simulink model "FAULT_MANAGEMENT"  (R2024b)
settings: configuration reference "MODEL_CONFIG_CHILD" (kept outside this file)
undefined symbols (not defined in the file): BATTERY_UV_LIM_U16, BATTERY_UV_RST_LIM_U16, BOOLEAN_ONE, CURR_CUTOFF_CTR_U16, CURRENTCUTOFF_LIM_mA_i32, DEFAULT_SPD_LIM_U16, MILLI_SEC_COUNTS_3000_U16, MILLI_SEC_COUNTS_5000_U16, MOTOR_BLOCK_CTR_U16, SAMPLE_TIME_1MS, THROTT_ERR_LWRTHSD_U16, THROTT_ERR_UPRTHSD_U16, THROTTLE_INITIATION_VALUE_U16, ZERO_i32, ZERO_U16
libraries: simulink x11
settings Model: DataDictionary=MCU_FOC_MAIN_DD.sldd  EnableAccessToBaseWorkspace=off  Creator=415  LastModifiedBy=415
settings ConfigSetRef: SourceName=MODEL_CONFIG_CHILD

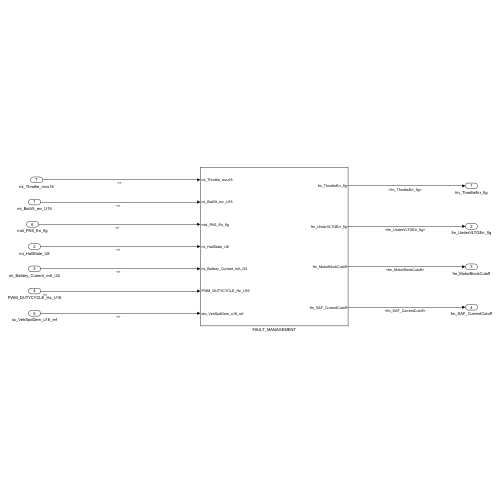
[thumbnail: Simulink's stored preview of the top-level diagram]
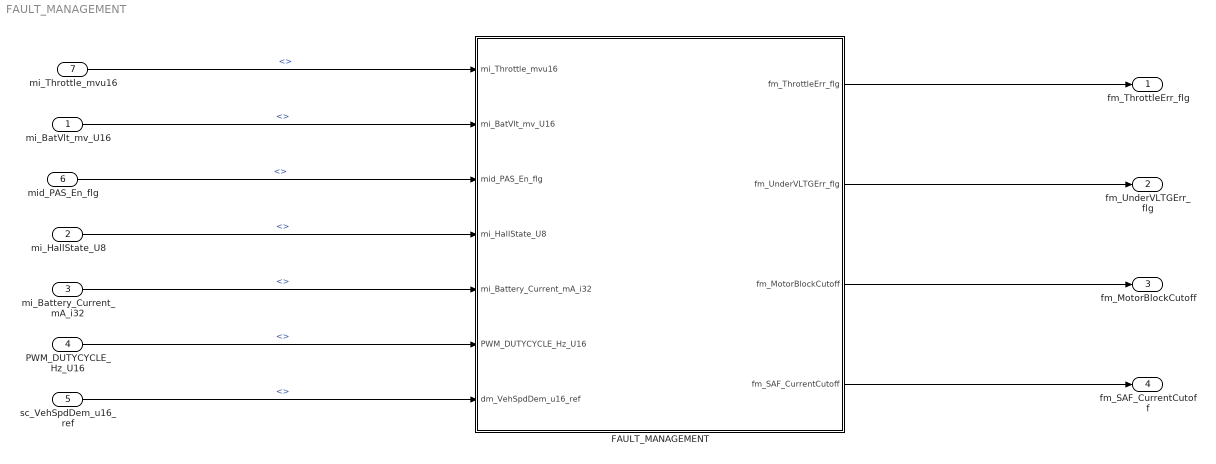
== system FAULT_MANAGEMENT ==
  mi_BatVlt_mv_U16 : Inport
  mi_HallState_U8 : Inport  Port=2
  mi_Battery_Current_mA_i32 : Inport  Port=3
  PWM_DUTYCYCLE_Hz_U16 : Inport  Port=4
  sc_VehSpdDem_u16_ref : Inport  Port=5
  mid_PAS_En_flg : Inport  Port=6
  mi_Throttle_mvu16 : Inport  Port=7
  FAULT_MANAGEMENT : Subsystem
  fm_ThrottleErr_flg : Outport
  fm_UnderVLTGErr_flg : Outport  Port=2
  fm_MotorBlockCutoff : Outport  Port=3
  fm_SAF_CurrentCutoff : Outport  Port=4
  wires:
  mi_Throttle_mvu16/1 -> FAULT_MANAGEMENT/1(mi_Throttle_mvu16)  "<>"
  sc_VehSpdDem_u16_ref/1 -> FAULT_MANAGEMENT/7(dm_VehSpdDem_u16_ref)  "<>"
  mi_BatVlt_mv_U16/1 -> FAULT_MANAGEMENT/2(mi_BatVlt_mv_U16)  "<>"
  FAULT_MANAGEMENT/1(fm_ThrottleErr_flg) -> fm_ThrottleErr_flg/1
  FAULT_MANAGEMENT/4(fm_SAF_CurrentCutoff) -> fm_SAF_CurrentCutoff/1
  mid_PAS_En_flg/1 -> FAULT_MANAGEMENT/3(mid_PAS_En_flg)  "<>"
  FAULT_MANAGEMENT/2(fm_UnderVLTGErr_flg) -> fm_UnderVLTGErr_flg/1
  FAULT_MANAGEMENT/3(fm_MotorBlockCutoff) -> fm_MotorBlockCutoff/1
  mi_Battery_Current_mA_i32/1 -> FAULT_MANAGEMENT/5(mi_Battery_Current_mA_i32)  "<>"
  PWM_DUTYCYCLE_Hz_U16/1 -> FAULT_MANAGEMENT/6(PWM_DUTYCYCLE_Hz_U16)  "<>"
  mi_HallState_U8/1 -> FAULT_MANAGEMENT/4(mi_HallState_U8)  "<>"

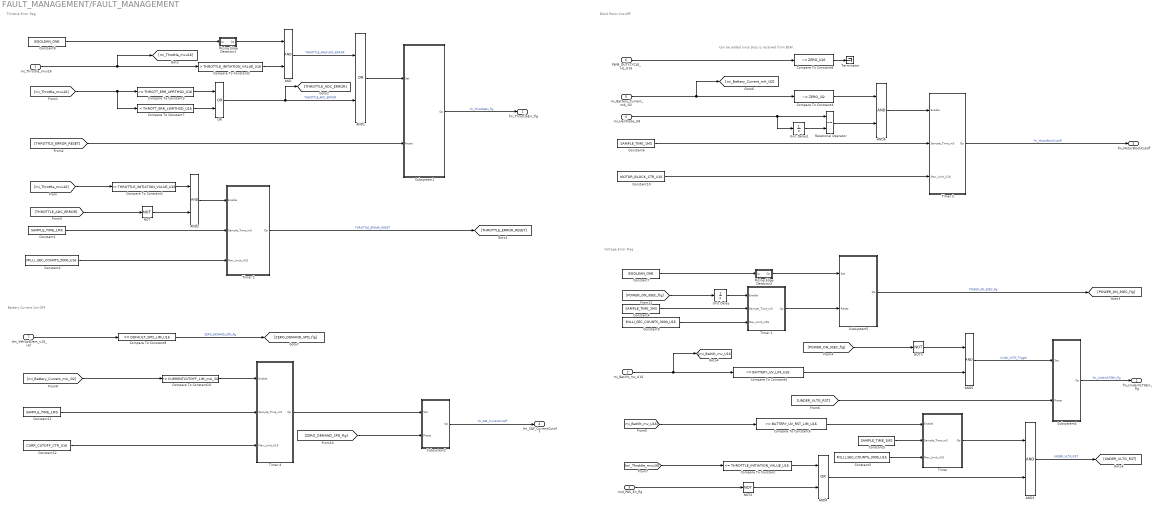
== system FAULT_MANAGEMENT/FAULT_MANAGEMENT ==
  note: Battery Current Cut-OFF
  note: Can be added once Duty is received from BSW.
  note: Block Rotor Cut-OFF
  note: Voltage Error Flag
  note: Throttle Error flag
  mi_Throttle_mvu16 : Inport
  mi_BatVlt_mv_U16 : Inport  Port=2
  mid_PAS_En_flg : Inport  Port=3
  mi_HallState_U8 : Inport  Port=4
  mi_Battery_Current_mA_i32 : Inport  Port=5
  PWM_DUTYCYCLE_Hz_U16 : Inport  Port=6
  dm_VehSpdDem_u16_ref : Inport  Port=7
  AND{,2..3,5..6} (5 alike) : Logic  AllPortsSameDT=off  OutDataTypeStr=boolean
  AND1 : Logic  Operator=OR  AllPortsSameDT=off  OutDataTypeStr=boolean
  AND4 : Logic  Operator=OR  AllPortsSameDT=off  OutDataTypeStr=boolean
  Compare To Constant : simulink/Logic and Bit Operations/Compare To Constant  relop=<=  const=THROTTLE_INITIATION_VALUE_U16  OutDataTypeStr=boolean
  Compare To Constant1 : simulink/Logic and Bit Operations/Compare To Constant  relop=<=  const=THROTTLE_INITIATION_VALUE_U16  OutDataTypeStr=boolean
  Compare To Constant10 : simulink/Logic and Bit Operations/Compare To Constant  relop=>=  const=CURRENTCUTOFF_LIM_mA_i32  OutDataTypeStr=boolean
  Compare To Constant2 : simulink/Logic and Bit Operations/Compare To Constant  relop=>  const=THROTTLE_INITIATION_VALUE_U16  OutDataTypeStr=boolean
  Compare To Constant3 : simulink/Logic and Bit Operations/Compare To Constant  relop=>=  const=THROTT_ERR_UPRTHSD_U16  OutDataTypeStr=boolean
  Compare To Constant4 : simulink/Logic and Bit Operations/Compare To Constant  relop=~=  const=ZERO_i32  OutDataTypeStr=boolean
  Compare To Constant5 : simulink/Logic and Bit Operations/Compare To Constant  relop=<=  const=BATTERY_UV_LIM_U16  OutDataTypeStr=boolean
  Compare To Constant6 : simulink/Logic and Bit Operations/Compare To Constant  relop=>=  const=BATTERY_UV_RST_LIM_U16  OutDataTypeStr=boolean
  Compare To Constant7 : simulink/Logic and Bit Operations/Compare To Constant  relop=<  const=THROTT_ERR_LWRTHSD_U16  OutDataTypeStr=boolean
  Compare To Constant8 : simulink/Logic and Bit Operations/Compare To Constant  relop=~=  const=ZERO_U16  OutDataTypeStr=boolean
  Compare To Constant9 : simulink/Logic and Bit Operations/Compare To Constant  relop===  const=DEFAULT_SPD_LIM_U16  OutDataTypeStr=boolean
  Constant{1,4..6,11} (5 alike) : Constant  Value=SAMPLE_TIME_1MS
  Constant10 : Constant  Value=MOTOR_BLOCK_CTR_U16
  Constant12 : Constant  Value=CURR_CUTOFF_CTR_U16
  Constant2 : Constant  Value=MILLI_SEC_COUNTS_5000_U16
  Constant3 : Constant  Value=MILLI_SEC_COUNTS_3000_U16
  Constant7 : Constant  Value=BOOLEAN_ONE
  Constant8 : Constant  Value=BOOLEAN_ONE
  Constant9 : Constant  Value=MILLI_SEC_COUNTS_3000_U16
  NOT : Logic  Operator=NOT  IconShape=distinctive  AllPortsSameDT=off  OutDataTypeStr=boolean
  NOT2 : Logic  Operator=NOT  IconShape=distinctive  AllPortsSameDT=off  OutDataTypeStr=boolean
  NOT3 : Logic  Operator=NOT  IconShape=distinctive  AllPortsSameDT=off  OutDataTypeStr=boolean
  OR : Logic  Operator=OR  AllPortsSameDT=off  OutDataTypeStr=boolean
  Relational Operator : RelationalOperator  Operator===  OutDataTypeStr=boolean  RndMeth=Simplest  InputSameDT=off
  Rising Edge Detector1 : Subsystem
  Rising Edge Detector2 : Subsystem
  Subsystem1 : Subsystem
  Subsystem2 : Subsystem
  Subsystem4 : Subsystem
  Subsystem5 : Subsystem
  Terminator : Terminator
  "Timer " : Subsystem
  Timer 1 : Subsystem
  Timer 2 : Subsystem
  Timer 3 : Subsystem
  Timer 4 : Subsystem
  Unit Delay : UnitDelay  SampleTime=-1  HasFrameUpgradeWarning=on
  Unit Delay1 : UnitDelay  SampleTime=-1  HasFrameUpgradeWarning=on
  fm_ThrottleErr_flg : Outport
  fm_UnderVLTGErr_flg : Outport  Port=2
  fm_MotorBlockCutoff : Outport  Port=3  OutputWhenDisabled=reset  InitialOutput=0
  fm_SAF_CurrentCutoff : Outport  Port=4  OutputWhenDisabled=reset  InitialOutput=0
  wires:
  Constant8/1 -> Rising Edge Detector1/1(Ip)
  mi_Throttle_mvu16/1 -> Compare To Constant2/1, [mi_Throttle_mvu16]
  Compare To Constant2/1 -> AND/2
  Rising Edge Detector1/1(Op) -> AND/1
  AND/1 -> AND1/1  "THROTTLE_MALFUNC_ERROR"
  Timer 2/1(Op) -> [THROTTLE_ERROR_RESET]  "THROTTLE_ERROR_RESET"
  Constant1/1 -> Timer 2/2(Sample_Time_mS)
  Compare To Constant1/1 -> AND2/1
  [mi_Throttle_mvu16] -> Compare To Constant1/1
  Constant2/1 -> Timer 2/3(Max_Limit_U16)
  Subsystem1/1(Op) -> fm_ThrottleErr_flg/1  "fm_ThrottleErr_flg"
  Compare To Constant7/1 -> OR/2
  Compare To Constant3/1 -> OR/1
  [THROTTLE_ERROR_RESET] -> Subsystem1/2(Reset)
  AND1/1 -> Subsystem1/1(Set)
  [mi_Throttle_mvu16] -> Compare To Constant3/1, Compare To Constant7/1
  OR/1 -> [THROTTLE_ADC_ERROR], AND1/2  "THROTTLE_ADC_ERROR"
  [THROTTLE_ADC_ERROR] -> NOT/1
  NOT/1 -> AND2/2
  AND2/1 -> Timer 2/1(Enable)
  Unit Delay/1 -> Timer 1/1(Enable)
  NOT3/1 -> AND5/1
  NOT2/1 -> AND4/2
  Subsystem5/1(Op) -> [POWER_ON_3SEC_flg]  "POWER_ON_3SEC_flg"
  Subsystem4/1(Op) -> fm_UnderVLTGErr_flg/1  "fm_UnderVLTGErr_flg"
  Compare To Constant5/1 -> AND5/2
  mid_PAS_En_flg/1 -> NOT2/1
  [mi_Throttle_mvu16] -> Compare To Constant/1
  Constant9/1 -> Timer 1/3(Max_Limit_U16)
  Constant4/1 -> Timer 1/2(Sample_Time_mS)
  Constant5/1 -> "Timer "/2(Sample_Time_mS)
  Rising Edge Detector2/1(Op) -> Subsystem5/1(Set)
  Compare To Constant6/1 -> "Timer "/1(Enable)
  Compare To Constant/1 -> AND4/1
  [POWER_ON_3SEC_flg] -> Unit Delay/1
  Constant7/1 -> Rising Edge Detector2/1(Ip)
  AND5/1 -> Subsystem4/1(Set)  "Under_VLTG_Trigger"
  mi_BatVlt_mv_U16/1 -> [mi_BatVlt_mv_U16], Compare To Constant5/1
  "Timer "/1(Op) -> AND3/1
  AND4/1 -> AND3/2
  Timer 1/1(Op) -> Subsystem5/2(Reset)
  [UNDER_VLTG_RST] -> Subsystem4/2(Reset)
  Constant3/1 -> "Timer "/3(Max_Limit_U16)
  [POWER_ON_3SEC_flg] -> NOT3/1
  [mi_BatVlt_mv_U16] -> Compare To Constant6/1
  AND3/1 -> [UNDER_VLTG_RST]  "UNDER_VLTG_RST"
  Timer 3/1(Op) -> fm_MotorBlockCutoff/1  "fm_MotorBlockCutoff"
  AND6/1 -> Timer 3/1(Enable)
  Relational Operator/1 -> AND6/2
  Compare To Constant4/1 -> AND6/1
  mi_Battery_Current_mA_i32/1 -> Compare To Constant4/1, [mi_Battery_Current_mA_i32]
  Unit Delay1/1 -> Relational Operator/2
  mi_HallState_U8/1 -> Unit Delay1/1, Relational Operator/1
  Constant6/1 -> Timer 3/2(Sample_Time_mS)
  Constant10/1 -> Timer 3/3(Max_Limit_U16)
  Compare To Constant8/1 -> Terminator/1
  PWM_DUTYCYCLE_Hz_U16/1 -> Compare To Constant8/1
  Constant11/1 -> Timer 4/2(Sample_Time_mS)
  Compare To Constant10/1 -> Timer 4/1(Enable)
  [mi_Battery_Current_mA_i32] -> Compare To Constant10/1
  Timer 4/1(Op) -> Subsystem2/1(Set)
  Constant12/1 -> Timer 4/3(Max_Limit_U16)
  dm_VehSpdDem_u16_ref/1 -> Compare To Constant9/1
  Compare To Constant9/1 -> [ZERO_DEMAND_SPD_flg]  "ZERO_DEMAND_SPD_flg"
  [ZERO_DEMAND_SPD_flg] -> Subsystem2/2(Reset)
  Subsystem2/1(Op) -> fm_SAF_CurrentCutoff/1  "fm_SAF_CurrentCutoff"

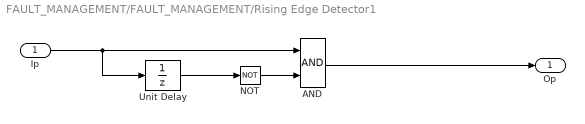
== system FAULT_MANAGEMENT/FAULT_MANAGEMENT/Rising Edge Detector1 ==
  Ip : Inport
  AND : Logic  AllPortsSameDT=off  OutDataTypeStr=boolean
  NOT : Logic  Operator=NOT  IconShape=distinctive  AllPortsSameDT=off  OutDataTypeStr=boolean
  Unit Delay : UnitDelay  SampleTime=-1  HasFrameUpgradeWarning=on
  Op : Outport
  wires:
  Unit Delay/1 -> NOT/1
  NOT/1 -> AND/2
  AND/1 -> Op/1
  Ip/1 -> AND/1, Unit Delay/1

== system FAULT_MANAGEMENT/FAULT_MANAGEMENT/Rising Edge Detector2 ==
  Ip : Inport
  AND : Logic  AllPortsSameDT=off  OutDataTypeStr=boolean
  NOT : Logic  Operator=NOT  IconShape=distinctive  AllPortsSameDT=off  OutDataTypeStr=boolean
  Unit Delay : UnitDelay  SampleTime=-1  HasFrameUpgradeWarning=on
  Op : Outport
  wires:
  Ip/1 -> Unit Delay/1, AND/1
  AND/1 -> Op/1
  NOT/1 -> AND/2
  Unit Delay/1 -> NOT/1

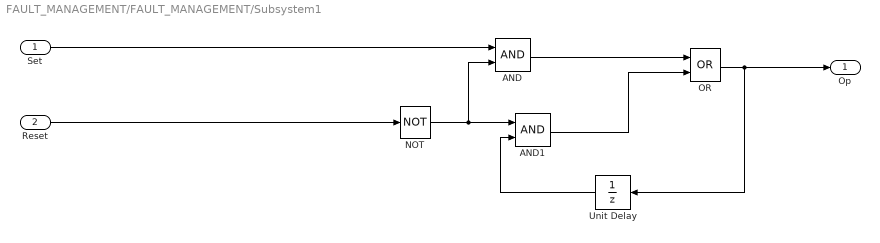
== system FAULT_MANAGEMENT/FAULT_MANAGEMENT/Subsystem1 ==
  Set : Inport
  Reset : Inport  Port=2
  AND : Logic  AllPortsSameDT=off  OutDataTypeStr=boolean
  AND1 : Logic  AllPortsSameDT=off  OutDataTypeStr=boolean
  NOT : Logic  Operator=NOT  IconShape=distinctive  AllPortsSameDT=off  OutDataTypeStr=boolean
  OR : Logic  Operator=OR  AllPortsSameDT=off  OutDataTypeStr=boolean
  Unit Delay : UnitDelay  SampleTime=-1  HasFrameUpgradeWarning=on
  Op : Outport
  wires:
  Reset/1 -> NOT/1
  OR/1 -> Unit Delay/1, Op/1
  NOT/1 -> AND1/1, AND/2
  Unit Delay/1 -> AND1/2
  Set/1 -> AND/1
  AND/1 -> OR/1
  AND1/1 -> OR/2

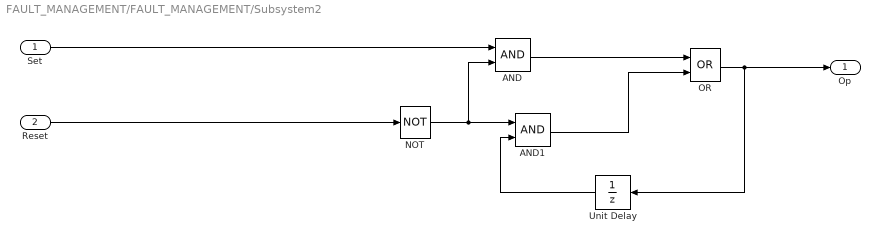
== system FAULT_MANAGEMENT/FAULT_MANAGEMENT/Subsystem2 ==
  Set : Inport
  Reset : Inport  Port=2
  AND : Logic  AllPortsSameDT=off  OutDataTypeStr=boolean
  AND1 : Logic  AllPortsSameDT=off  OutDataTypeStr=boolean
  NOT : Logic  Operator=NOT  IconShape=distinctive  AllPortsSameDT=off  OutDataTypeStr=boolean
  OR : Logic  Operator=OR  AllPortsSameDT=off  OutDataTypeStr=boolean
  Unit Delay : UnitDelay  SampleTime=-1  HasFrameUpgradeWarning=on
  Op : Outport
  wires:
  AND1/1 -> OR/2
  AND/1 -> OR/1
  Set/1 -> AND/1
  Unit Delay/1 -> AND1/2
  NOT/1 -> AND/2, AND1/1
  OR/1 -> Op/1, Unit Delay/1
  Reset/1 -> NOT/1

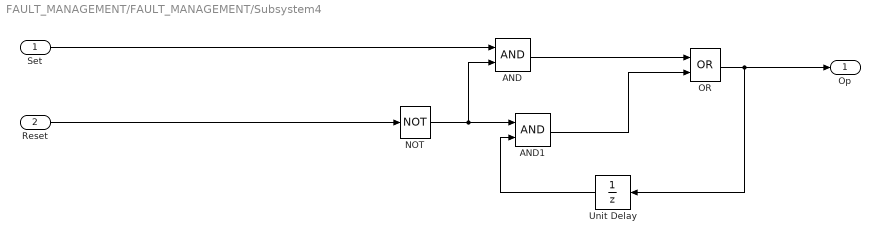
== system FAULT_MANAGEMENT/FAULT_MANAGEMENT/Subsystem4 ==
  Set : Inport
  Reset : Inport  Port=2
  AND : Logic  AllPortsSameDT=off  OutDataTypeStr=boolean
  AND1 : Logic  AllPortsSameDT=off  OutDataTypeStr=boolean
  NOT : Logic  Operator=NOT  IconShape=distinctive  AllPortsSameDT=off  OutDataTypeStr=boolean
  OR : Logic  Operator=OR  AllPortsSameDT=off  OutDataTypeStr=boolean
  Unit Delay : UnitDelay  SampleTime=-1  HasFrameUpgradeWarning=on
  Op : Outport
  wires:
  AND1/1 -> OR/2
  AND/1 -> OR/1
  Set/1 -> AND/1
  Unit Delay/1 -> AND1/2
  NOT/1 -> AND/2, AND1/1
  OR/1 -> Op/1, Unit Delay/1
  Reset/1 -> NOT/1

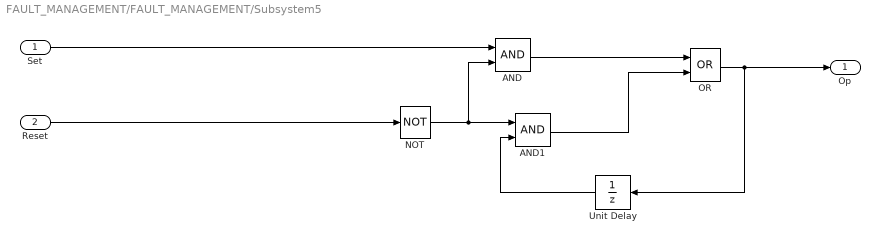
== system FAULT_MANAGEMENT/FAULT_MANAGEMENT/Subsystem5 ==
  Set : Inport
  Reset : Inport  Port=2
  AND : Logic  AllPortsSameDT=off  OutDataTypeStr=boolean
  AND1 : Logic  AllPortsSameDT=off  OutDataTypeStr=boolean
  NOT : Logic  Operator=NOT  IconShape=distinctive  AllPortsSameDT=off  OutDataTypeStr=boolean
  OR : Logic  Operator=OR  AllPortsSameDT=off  OutDataTypeStr=boolean
  Unit Delay : UnitDelay  SampleTime=-1  HasFrameUpgradeWarning=on
  Op : Outport
  wires:
  Reset/1 -> NOT/1
  OR/1 -> Unit Delay/1, Op/1
  NOT/1 -> AND1/1, AND/2
  Unit Delay/1 -> AND1/2
  Set/1 -> AND/1
  AND/1 -> OR/1
  AND1/1 -> OR/2

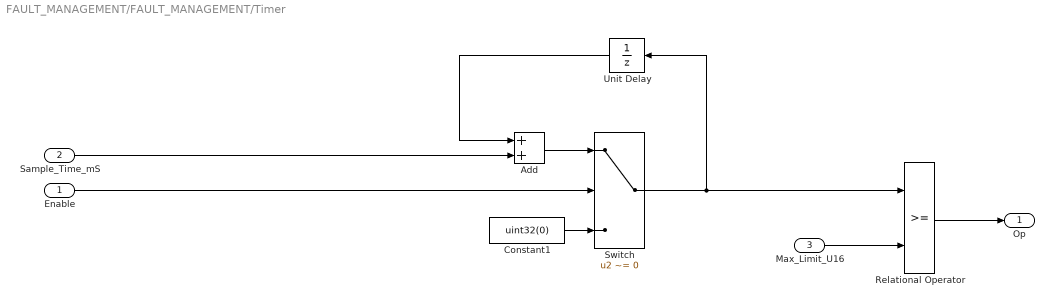
== system FAULT_MANAGEMENT/FAULT_MANAGEMENT/Timer  ==
  Enable : Inport
  Sample_Time_mS : Inport  Port=2
  Max_Limit_U16 : Inport  Port=3
  Add : Sum
  Constant1 : Constant  Value=uint32(0)
  Relational Operator : RelationalOperator  OutDataTypeStr=boolean  RndMeth=Simplest  InputSameDT=off
  Switch : Switch  Criteria=u2 ~= 0  SaturateOnIntegerOverflow=off  InputSameDT=off
  Unit Delay : UnitDelay  SampleTime=-1  HasFrameUpgradeWarning=on
  Op : Outport
  wires:
  Max_Limit_U16/1 -> Relational Operator/2
  Relational Operator/1 -> Op/1
  Enable/1 -> Switch/2
  Constant1/1 -> Switch/3
  Add/1 -> Switch/1
  Sample_Time_mS/1 -> Add/2
  Unit Delay/1 -> Add/1
  Switch/1 -> Relational Operator/1, Unit Delay/1

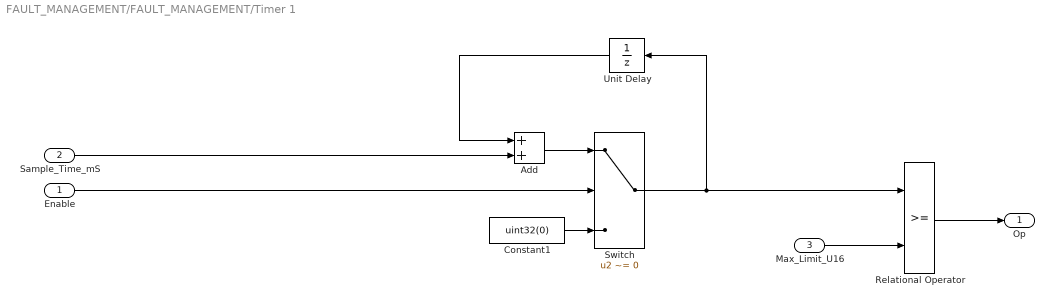
== system FAULT_MANAGEMENT/FAULT_MANAGEMENT/Timer 1 ==
  Enable : Inport
  Sample_Time_mS : Inport  Port=2
  Max_Limit_U16 : Inport  Port=3
  Add : Sum
  Constant1 : Constant  Value=uint32(0)
  Relational Operator : RelationalOperator  OutDataTypeStr=boolean  RndMeth=Simplest  InputSameDT=off
  Switch : Switch  Criteria=u2 ~= 0  SaturateOnIntegerOverflow=off  InputSameDT=off
  Unit Delay : UnitDelay  SampleTime=-1  HasFrameUpgradeWarning=on
  Op : Outport
  wires:
  Switch/1 -> Unit Delay/1, Relational Operator/1
  Unit Delay/1 -> Add/1
  Sample_Time_mS/1 -> Add/2
  Add/1 -> Switch/1
  Constant1/1 -> Switch/3
  Enable/1 -> Switch/2
  Relational Operator/1 -> Op/1
  Max_Limit_U16/1 -> Relational Operator/2

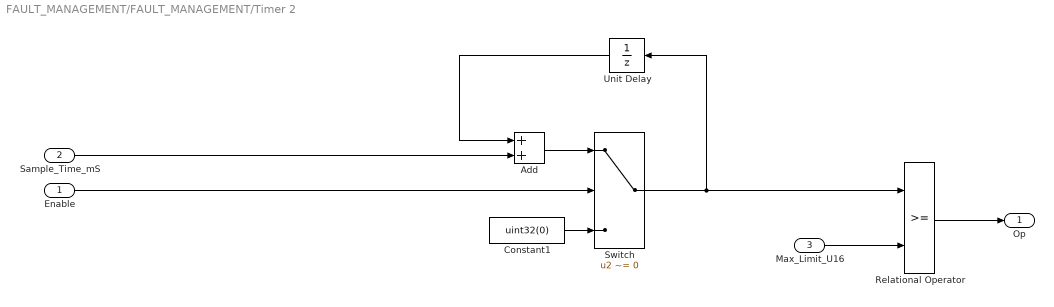
== system FAULT_MANAGEMENT/FAULT_MANAGEMENT/Timer 2 ==
  Enable : Inport
  Sample_Time_mS : Inport  Port=2
  Max_Limit_U16 : Inport  Port=3
  Add : Sum
  Constant1 : Constant  Value=uint32(0)
  Relational Operator : RelationalOperator  OutDataTypeStr=boolean  RndMeth=Simplest  InputSameDT=off
  Switch : Switch  Criteria=u2 ~= 0  SaturateOnIntegerOverflow=off  InputSameDT=off
  Unit Delay : UnitDelay  SampleTime=-1  HasFrameUpgradeWarning=on
  Op : Outport
  wires:
  Max_Limit_U16/1 -> Relational Operator/2
  Relational Operator/1 -> Op/1
  Enable/1 -> Switch/2
  Constant1/1 -> Switch/3
  Add/1 -> Switch/1
  Sample_Time_mS/1 -> Add/2
  Unit Delay/1 -> Add/1
  Switch/1 -> Relational Operator/1, Unit Delay/1

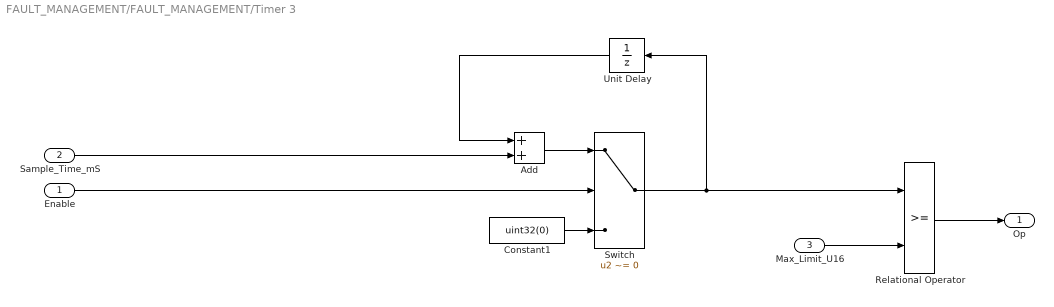
== system FAULT_MANAGEMENT/FAULT_MANAGEMENT/Timer 3 ==
  Enable : Inport
  Sample_Time_mS : Inport  Port=2
  Max_Limit_U16 : Inport  Port=3
  Add : Sum
  Constant1 : Constant  Value=uint32(0)
  Relational Operator : RelationalOperator  OutDataTypeStr=boolean  RndMeth=Simplest  InputSameDT=off
  Switch : Switch  Criteria=u2 ~= 0  SaturateOnIntegerOverflow=off  InputSameDT=off
  Unit Delay : UnitDelay  SampleTime=-1  HasFrameUpgradeWarning=on
  Op : Outport
  wires:
  Switch/1 -> Unit Delay/1, Relational Operator/1
  Unit Delay/1 -> Add/1
  Sample_Time_mS/1 -> Add/2
  Add/1 -> Switch/1
  Constant1/1 -> Switch/3
  Enable/1 -> Switch/2
  Relational Operator/1 -> Op/1
  Max_Limit_U16/1 -> Relational Operator/2

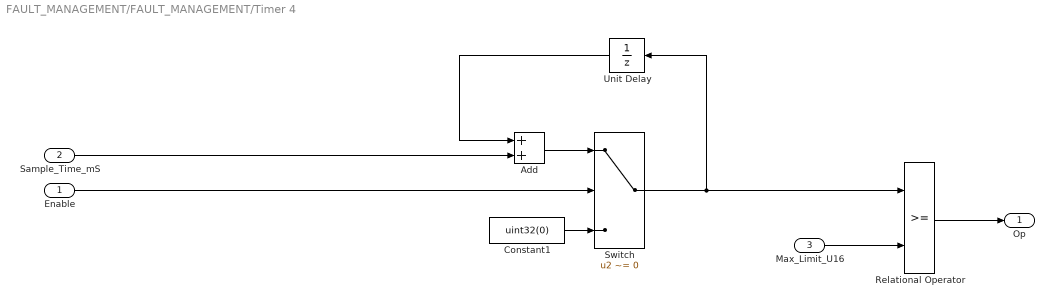
== system FAULT_MANAGEMENT/FAULT_MANAGEMENT/Timer 4 ==
  Enable : Inport
  Sample_Time_mS : Inport  Port=2
  Max_Limit_U16 : Inport  Port=3
  Add : Sum
  Constant1 : Constant  Value=uint32(0)
  Relational Operator : RelationalOperator  OutDataTypeStr=boolean  RndMeth=Simplest  InputSameDT=off
  Switch : Switch  Criteria=u2 ~= 0  SaturateOnIntegerOverflow=off  InputSameDT=off
  Unit Delay : UnitDelay  SampleTime=-1  HasFrameUpgradeWarning=on
  Op : Outport
  wires:
  Max_Limit_U16/1 -> Relational Operator/2
  Relational Operator/1 -> Op/1
  Enable/1 -> Switch/2
  Constant1/1 -> Switch/3
  Add/1 -> Switch/1
  Sample_Time_mS/1 -> Add/2
  Unit Delay/1 -> Add/1
  Switch/1 -> Relational Operator/1, Unit Delay/1
